simulink model "seed"  (R2024b)
settings: Solver=VariableStepAuto  StartTime=0.0  StopTime=10  RelTol=1e-3
values from neighbouring files (symbols this model uses):
  k = 0.41    [seedlab.m]
  kp = 10    [seedlab.m]
  sigma = 0.345    [seedlab.m]
libraries: simulink x1
settings Model: Creator=caleb  LastModifiedBy=caleb

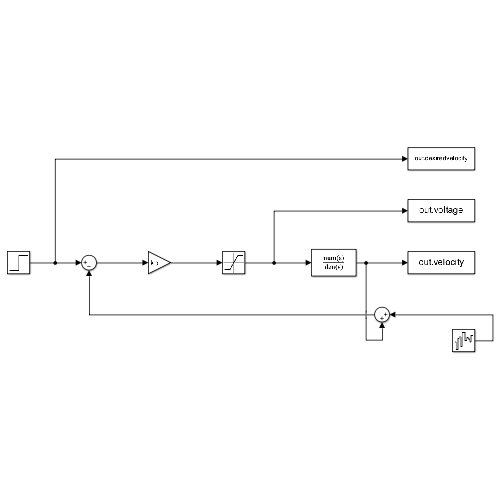
[thumbnail: Simulink's stored preview of the top-level diagram]
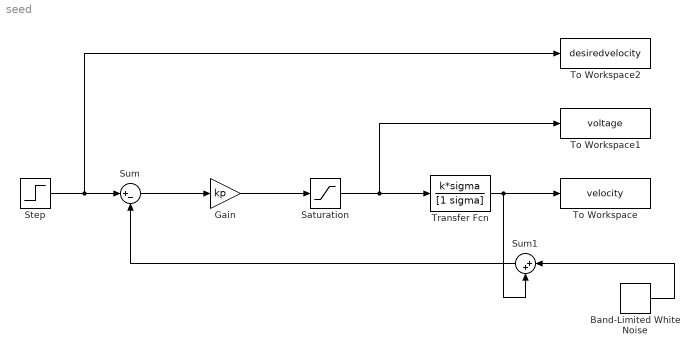
== system seed ==
  Band-Limited White Noise : simulink/Sources/Band-Limited White Noise  Cov=[0.0001]  Ts=0.001  seed=[23341]
  Gain : Gain  Gain=kp
  Saturation : Saturate  UpperLimit=7.5  LowerLimit=-7.5
  Step : Step  After=0.35  SampleTime=0
  Sum : Sum  Inputs=|+-
  Sum1 : Sum  Inputs=|++
  To Workspace : ToWorkspace  VariableName=velocity  SaveFormat=Timeseries  SampleTime=-1
  To Workspace1 : ToWorkspace  VariableName=voltage  SaveFormat=Timeseries  SampleTime=-1
  To Workspace2 : ToWorkspace  VariableName=desiredvelocity  SaveFormat=Timeseries  SampleTime=-1
  Transfer Fcn : TransferFcn  Numerator=k*sigma  Denominator=[1 sigma]
  wires:
  Step/1 -> To Workspace2/1, Sum/1
  Sum/1 -> Gain/1
  Gain/1 -> Saturation/1
  Saturation/1 -> Transfer Fcn/1, To Workspace1/1
  Transfer Fcn/1 -> To Workspace/1, Sum1/2
  Band-Limited White Noise/1 -> Sum1/1
  Sum1/1 -> Sum/2
